simulink model "forcetosbcomm"  (R2014a)
settings: Solver=ode3  StartTime=0.0  StopTime=inf  FixedStep=0.001  RelTol=1e-3
undefined symbols (not defined in the file): simget
libraries: jr3lib x2, rtai_utilities x1, sfbc_lib x1
settings Model: Creator=wirnshofer  LastModifiedBy=bschmidt
settings DataIOCC: SignalLoggingSaveFormat=ModelDataLogs
settings RTWCC: SystemTargetFile=prt.tlc  TemplateMakefile=prt.tmf  Description=Linux PREEMPT_RT Real-Time Target  ProcessScript=prt_make_rtw_hook
settings STFCustomTargetCC: TargetLangStandard=C99 (ISO)  CodeReplacementLibrary=GNU C99 extensions  ModelReferenceCompliant=off  ConcurrentExecutionCompliant=off  MatFileLogging=on  SystemTargetFile=prt.tlc
settings GRTTargetCC: TargetLangStandard=C99 (ISO)  CodeReplacementLibrary=GNU C99 extensions  ModelReferenceCompliant=off  ParMdlRefBuildCompliant=off  CompOptLevelCompliant=off  ConcurrentExecutionCompliant=off  CombineOutputUpdateFcns=off  CPPClassGenCompliant=off  GRTInterface=on

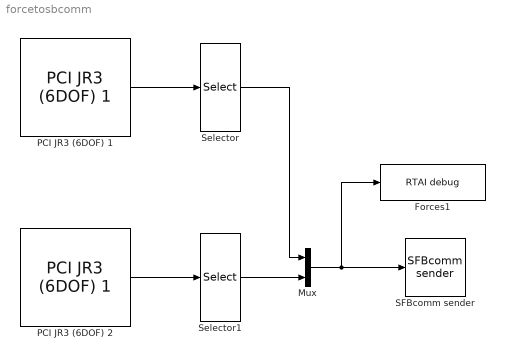
== system forcetosbcomm ==
  Forces1 : rtai_utilities/RTAI debug  rate=1
  Mux : Mux  Inputs=2
  PCI JR3 (6DOF) 1 : jr3lib/PCI JR3 (6DOF) 1  bd_number=0  filter_nr=1  sampletime=simget(bdroot,'FixedStep')  begin_reset=on
  PCI JR3 (6DOF) 2 : jr3lib/PCI JR3 (6DOF) 1  bd_number=1  filter_nr=1  sampletime=simget(bdroot,'FixedStep')  begin_reset=on
  SFBcomm sender : sfbc_lib/SFBcomm sender  localPort=11112  streamID=1  portNames=A  connectTimeout=200  sampleTime=-1
  Selector : Selector  InputPortWidth=6  Indices=[1 2 3]
  Selector1 : Selector  InputPortWidth=6  Indices=[1 2 3]
  wires:
  PCI JR3 (6DOF) 1/1 -> Selector/1
  PCI JR3 (6DOF) 2/1 -> Selector1/1
  Mux/1 -> Forces1/1, SFBcomm sender/1
  Selector1/1 -> Mux/2
  Selector/1 -> Mux/1
